simulink model "distiller"  (R2016b)
settings: Solver=VariableStepAuto  StartTime=0.0  StopTime=10.0  RelTol=1e-3
settings Model: Creator=rjg01  LastModifiedBy=rjg01

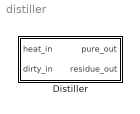
== system distiller ==
  Distiller : Subsystem

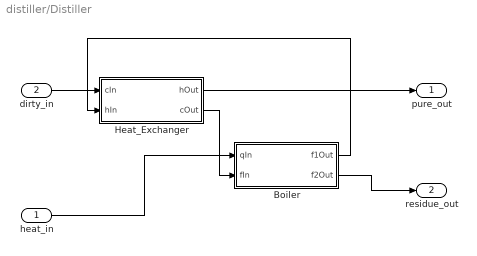
== system distiller/Distiller ==
  heat_in : Inport  OutDataTypeStr=Bus: Heat
  "dirty_in " : Inport  Port=2  OutDataTypeStr=Bus: Fluid
  "Boiler " : Subsystem
  Heat_Exchanger : Subsystem
  pure_out : Outport  OutDataTypeStr=Bus: Fluid
  residue_out : Outport  Port=2  OutDataTypeStr=Bus: Fluid
  wires:
  "dirty_in "/1 -> Heat_Exchanger/1(cIn)
  Heat_Exchanger/1(hOut) -> pure_out/1
  heat_in/1 -> "Boiler "/1(qIn)
  Heat_Exchanger/2("cOut ") -> "Boiler "/2("fIn ")
  "Boiler "/2(f2Out) -> residue_out/1
  "Boiler "/1(f1Out) -> Heat_Exchanger/2(hIn)

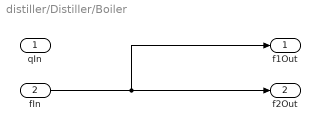
== system distiller/Distiller/Boiler  ==
  qIn : Inport  OutDataTypeStr=Bus: Heat
  "fIn " : Inport  Port=2  OutDataTypeStr=Bus: Fluid
  f1Out : Outport  OutDataTypeStr=Bus: Fluid
  f2Out : Outport  Port=2  OutDataTypeStr=Bus: Fluid
  wires:
  "fIn "/1 -> f1Out/1, f2Out/1

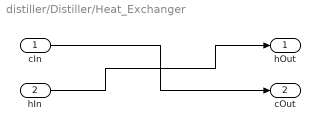
== system distiller/Distiller/Heat_Exchanger ==
  cIn : Inport  OutDataTypeStr=Bus: Fluid
  hIn : Inport  Port=2  OutDataTypeStr=Bus: Fluid
  hOut : Outport  OutDataTypeStr=Bus: Fluid
  "cOut " : Outport  Port=2  OutDataTypeStr=Bus: Fluid
  wires:
  cIn/1 -> "cOut "/1
  hIn/1 -> hOut/1
